simulink model "Ident_Validacao"  (R2015a)
settings: Solver=ode45  StartTime=0.0  StopTime=t(end)  RelTol=1e-3
values from neighbouring files (symbols this model uses):
  T = 0.04    [Ident_RLtool.m]
  Y1 = tf( [3.48e-6 1.6 6.079], [1 -0.2635 0.007111 0.009379], T )    [Ident_RLtool.m]
  Y2 = tf( [0.0003065 2.198 5.651], [1 -0.3892 0.1132 -0.03574], T )    [Ident_RLtool.m]
  Y3 = tf( [-1.216e-06 2.3 6.046], [1 -0.2409 -0.004502 0.01131], T )    [Ident_RLtool.m]
  Y4 = tf( [0.001266 1.892 6.116], [1 -0.3787 0.0893 -0.04015 ], T )    [Ident_RLtool.m]
  Y5 = tf( [0.003993 0.4917 6.77 4.861], [1 0.3475 -0.08834 -0.1231 0.08894], T )    [Ident_RLtool.m]
settings Model: Creator=Lucas  LastModifiedBy=Lucas

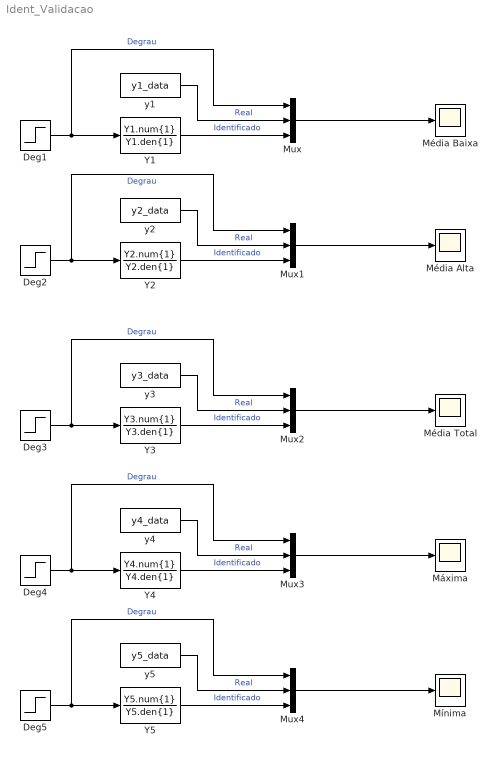
== system Ident_Validacao ==
  Deg{1..5} (5 alike) : Step  Time=6*T  After=10  SampleTime=T
  Mux{,1..4} (5 alike) : Mux  Inputs=3
  Máxima : Scope
      settings: ShowLegends=on  SaveName=ScopeData3
  Média Alta : Scope
      settings: ShowLegends=on  SaveName=ScopeData2
  "Média Baixa " : Scope
      settings: ShowLegends=on
  Média Total : Scope
      settings: ShowLegends=on
  Mínima : Scope
      settings: ShowLegends=on  SaveName=ScopeData4
  Y1 : DiscreteTransferFcn  Numerator=Y1.num{1}  Denominator=Y1.den{1}  SampleTime=T
  Y2 : DiscreteTransferFcn  Numerator=Y2.num{1}  Denominator=Y2.den{1}  SampleTime=T
  Y3 : DiscreteTransferFcn  Numerator=Y3.num{1}  Denominator=Y3.den{1}  SampleTime=T
  Y4 : DiscreteTransferFcn  Numerator=Y4.num{1}  Denominator=Y4.den{1}  SampleTime=T
  Y5 : DiscreteTransferFcn  Numerator=Y5.num{1}  Denominator=Y5.den{1}  SampleTime=T
  y1 : FromWorkspace  VariableName=y1_data  SampleTime=T
  y2 : FromWorkspace  VariableName=y2_data  SampleTime=T
  y3 : FromWorkspace  VariableName=y3_data  SampleTime=T
  y4 : FromWorkspace  VariableName=y4_data  SampleTime=T
  y5 : FromWorkspace  VariableName=y5_data  SampleTime=T
  wires:
  Mux/1 -> "Média Baixa "/1
  Y1/1 -> Mux/3  "Identificado"
  Deg1/1 -> Mux/1, Y1/1  "Degrau"
  y1/1 -> Mux/2  "Real"
  Y2/1 -> Mux1/3  "Identificado"
  Deg2/1 -> Y2/1, Mux1/1  "Degrau"
  y2/1 -> Mux1/2  "Real"
  Y3/1 -> Mux2/3  "Identificado"
  Deg3/1 -> Mux2/1, Y3/1  "Degrau"
  y3/1 -> Mux2/2  "Real"
  Mux2/1 -> Média Total/1
  Mux1/1 -> Média Alta/1
  Y4/1 -> Mux3/3  "Identificado"
  Deg4/1 -> Y4/1, Mux3/1  "Degrau"
  y4/1 -> Mux3/2  "Real"
  Mux3/1 -> Máxima/1
  Y5/1 -> Mux4/3  "Identificado"
  Deg5/1 -> Mux4/1, Y5/1  "Degrau"
  y5/1 -> Mux4/2  "Real"
  Mux4/1 -> Mínima/1
